simulink model "mcp"  (R2020a)
settings: configuration reference "globalConfig" (kept outside this file)
InitFcn:
  | load pot.mat;
  | load rpm.mat;
undefined symbols (not defined in the file): pot_kw, rpm
settings Model: OrderedModelArguments=off  Creator=victo  LastModifiedBy=ToT_IPMS_03
settings ConfigSetRef: SourceName=globalConfig  SourceLocation=Base Workspace

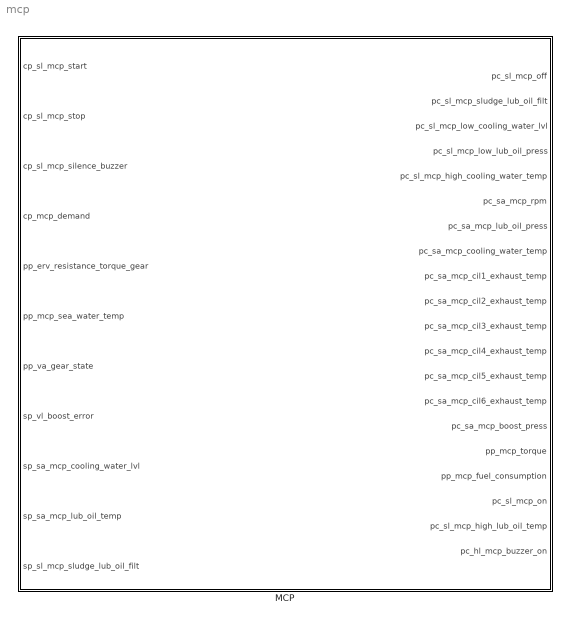
== system mcp ==
  MCP : Subsystem

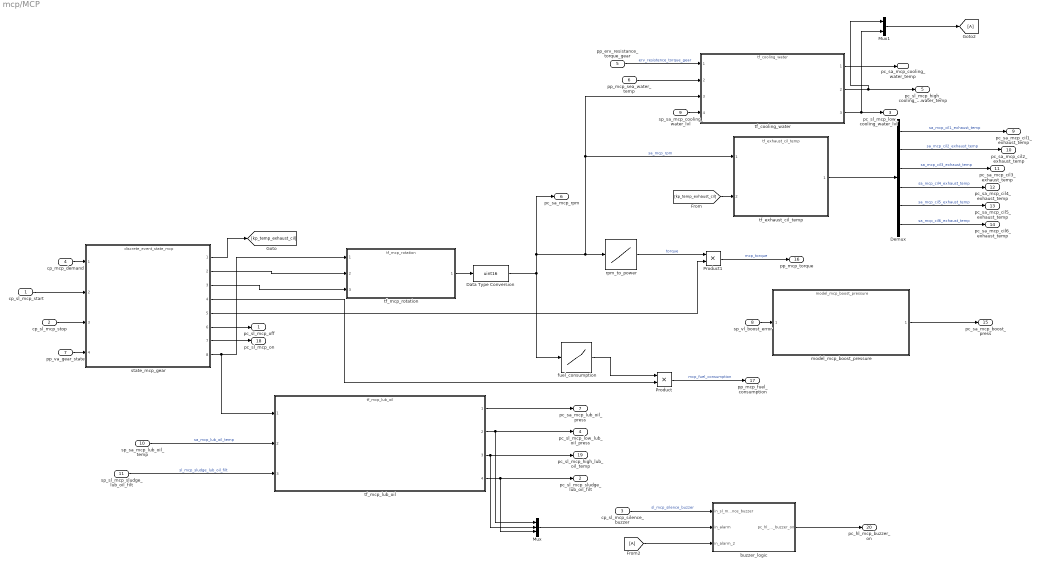
== system mcp/MCP ==
  cp_sl_mcp_start : Inport  OutMin=[0]  OutMax=[1]  OutDataTypeStr=boolean
  cp_sl_mcp_stop : Inport  Port=2  OutMin=[0]  OutMax=[1]  OutDataTypeStr=boolean
  cp_sl_mcp_silence_buzzer : Inport  Port=3  OutMin=[0]  OutMax=[1]  OutDataTypeStr=boolean
  cp_mcp_demand : Inport  Port=4  OutMin=[-100]  OutMax=[100]  OutDataTypeStr=int16  Unit=%
  pp_erv_resistance_torque_gear : Inport  Port=5  OutMin=0  OutMax=1000  OutDataTypeStr=double  Unit=N*m
  pp_mcp_sea_water_temp : Inport  Port=6  OutMin=0  OutMax=90  OutDataTypeStr=uint16  Unit=°C
  pp_va_gear_state : Inport  Port=7  OutMin=0  OutMax=2  OutDataTypeStr=uint8
  sp_vl_boost_error : Inport  Port=8  OutDataTypeStr=boolean
  sp_sa_mcp_cooling_water_lvl : Inport  Port=9  OutMin=[0]  OutMax=[100]  OutDataTypeStr=uint16  Unit=%
  sp_sa_mcp_lub_oil_temp : Inport  Port=10  OutMin=[0]  OutMax=[100]  OutDataTypeStr=uint16  Unit=°C
  sp_sl_mcp_sludge_lub_oil_filt : Inport  Port=11  OutDataTypeStr=boolean
  Data Type Conversion : DataTypeConversion  OutDataTypeStr=uint16
  Demux : Demux  Outputs=6
  Mux : Mux  Inputs=3
  Mux1 : Mux  Inputs=2
  Product : Product
  Product1 : Product
  buzzer_logic : Subsystem
  fuel_consumption : Lookup_n-D  NumberOfTableDimensions=1  BreakpointsForDimension1=[1000,1100,1200,1300,1400,1500,1600,1700,1800,1900]  Table=[25,30,37,45,55,68,82,101,122,145]  ExtrapMethod=Clip  InternalRulePriority=Speed  RndMeth=Simplest  InputSameDT=on
  model_mcp_boost_pressure : ModelReference  ModelNameDialog=model_mcp_boost_pressure  SimulationMode=Normal  ModelReferenceVersion=2.63
  rpm_to_power : Lookup_n-D  NumberOfTableDimensions=1  BreakpointsForDimension1=rpm  Table=pot_kw./rpm  ExtrapMethod=Clip  InternalRulePriority=Speed  RndMeth=Simplest  InputSameDT=on
  state_mcp_gear : ModelReference  ModelNameDialog=discrete_event_state_mcp.slx  SimulationMode=Normal  ModelReferenceVersion=2.44
  tf_cooling_water : ModelReference  ModelNameDialog=tf_cooling_water.slx  SimulationMode=Normal  ModelReferenceVersion=1.16
  tf_exhaust_cil_temp : ModelReference  ModelNameDialog=tf_exhaust_cil_temp.slx  SimulationMode=Normal  ModelReferenceVersion=1.10
  tf_mcp_lub_oil : ModelReference  ModelNameDialog=tf_mcp_lub_oil  SimulationMode=Normal  ModelReferenceVersion=1.29
  tf_mcp_rotation : ModelReference  ModelNameDialog=tf_mcp_rotation.slx  SimulationMode=Normal  ModelReferenceVersion=2.30
  pc_sl_mcp_off : Outport  OutMin=[0]  OutMax=[1]  OutDataTypeStr=boolean
  pc_sl_mcp_sludge_lub_oil_filt : Outport  Port=2  OutMin=[0]  OutMax=[1]  OutDataTypeStr=boolean
  pc_sl_mcp_low_cooling_water_lvl : Outport  Port=3  OutMin=[0]  OutMax=[1]  OutDataTypeStr=boolean
  pc_sl_mcp_low_lub_oil_press : Outport  Port=4  OutMin=[0]  OutMax=[1]  OutDataTypeStr=boolean
  pc_sl_mcp_high_cooling_water_temp : Outport  Port=5  OutMin=[0]  OutMax=[1]  OutDataTypeStr=boolean
  pc_sa_mcp_rpm : Outport  Port=6  OutMin=[0]  OutMax=[2000]  OutDataTypeStr=uint16  Unit=rpm
  pc_sa_mcp_lub_oil_press : Outport  Port=7  OutMin=[0]  OutMax=[100]  OutDataTypeStr=uint16  Unit=MPa
  pc_sa_mcp_cooling_water_temp : Outport  Port=8  OutMin=[0]  OutMax=[90]  OutDataTypeStr=uint16  Unit=°C
  pc_sa_mcp_cil1_exhaust_temp : Outport  Port=9  OutMin=[20]  OutMax=[650]  OutDataTypeStr=uint16  Unit=°C
  pc_sa_mcp_cil2_exhaust_temp : Outport  Port=10  OutMin=[20]  OutMax=[650]  OutDataTypeStr=uint16  Unit=°C
  pc_sa_mcp_cil3_exhaust_temp : Outport  Port=11  OutMin=[20]  OutMax=[650]  OutDataTypeStr=uint16  Unit=°C
  pc_sa_mcp_cil4_exhaust_temp : Outport  Port=12  OutMin=[20]  OutMax=[650]  OutDataTypeStr=uint16  Unit=°C
  pc_sa_mcp_cil5_exhaust_temp : Outport  Port=13  OutMin=[20]  OutMax=[650]  OutDataTypeStr=uint16  Unit=°C
  pc_sa_mcp_cil6_exhaust_temp : Outport  Port=14  OutMin=[20]  OutMax=[650]  OutDataTypeStr=uint16  Unit=°C
  pc_sa_mcp_boost_press : Outport  Port=15  OutMin=[-10]  OutMax=[10]  OutDataTypeStr=int16  Unit=MPa
  pp_mcp_torque : Outport  Port=16
  pp_mcp_fuel_consumption : Outport  Port=17
  pc_sl_mcp_on : Outport  Port=18  OutMin=[0]  OutMax=[1]  OutDataTypeStr=boolean
  pc_sl_mcp_high_lub_oil_temp : Outport  Port=19  OutDataTypeStr=boolean
  pc_hl_mcp_buzzer_on : Outport  Port=20
  wires:
  cp_mcp_demand/1 -> state_mcp_gear/1
  tf_mcp_rotation/1 -> Data Type Conversion/1
  tf_mcp_lub_oil/1 -> pc_sa_mcp_lub_oil_press/1
  fuel_consumption/1 -> Product/1
  Product/1 -> pp_mcp_fuel_consumption/1  "mcp_fuel_consumption"
  rpm_to_power/1 -> Product1/1  "torque"
  Product1/1 -> pp_mcp_torque/1  "mcp_torque"
  Demux/1 -> pc_sa_mcp_cil1_exhaust_temp/1  "sa_mcp_cil1_exhaust_temp"
  Demux/2 -> pc_sa_mcp_cil2_exhaust_temp/1  "sa_mcp_cil2_exhaust_temp"
  Demux/3 -> pc_sa_mcp_cil3_exhaust_temp/1  "sa_mcp_cil3_exhaust_temp"
  Demux/4 -> pc_sa_mcp_cil4_exhaust_temp/1  "sa_mcp_cil4_exhaust_temp"
  Demux/5 -> pc_sa_mcp_cil5_exhaust_temp/1  "sa_mcp_cil5_exhaust_temp"
  Demux/6 -> pc_sa_mcp_cil6_exhaust_temp/1  "sa_mcp_cil6_exhaust_temp"
  [kp_temp_exhaust_cil] -> tf_exhaust_cil_temp/2
  tf_exhaust_cil_temp/1 -> Demux/1
  cp_sl_mcp_stop/1 -> state_mcp_gear/3
  state_mcp_gear/1 -> [kp_temp_exhaust_cil]
  state_mcp_gear/2 -> tf_mcp_rotation/2
  state_mcp_gear/3 -> tf_mcp_rotation/3
  state_mcp_gear/4 -> Product/2
  state_mcp_gear/5 -> Product1/2
  state_mcp_gear/6 -> pc_sl_mcp_off/1
  state_mcp_gear/7 -> pc_sl_mcp_on/1
  pp_mcp_sea_water_temp/1 -> tf_cooling_water/2
  pp_erv_resistance_torque_gear/1 -> tf_cooling_water/1  "erv_resistence_torque_gear"
  tf_cooling_water/1 -> pc_sa_mcp_cooling_water_temp/1
  state_mcp_gear/8 -> tf_mcp_lub_oil/1, tf_mcp_rotation/1
  pp_va_gear_state/1 -> state_mcp_gear/4
  sp_vl_boost_error/1 -> model_mcp_boost_pressure/1
  model_mcp_boost_pressure/1 -> pc_sa_mcp_boost_press/1
  Data Type Conversion/1 -> fuel_consumption/1, pc_sa_mcp_rpm/1, rpm_to_power/1, tf_exhaust_cil_temp/1, tf_cooling_water/3  "sa_mcp_rpm"
  sp_sa_mcp_cooling_water_lvl/1 -> tf_cooling_water/4
  tf_mcp_lub_oil/2 -> Mux/1, pc_sl_mcp_low_lub_oil_press/1
  sp_sa_mcp_lub_oil_temp/1 -> tf_mcp_lub_oil/2  "sa_mcp_lub_oil_temp"
  tf_mcp_lub_oil/3 -> Mux/2, pc_sl_mcp_high_lub_oil_temp/1
  sp_sl_mcp_sludge_lub_oil_filt/1 -> tf_mcp_lub_oil/3  "sl_mcp_sludge_lub_oil_filt"
  tf_mcp_lub_oil/4 -> Mux/3, pc_sl_mcp_sludge_lub_oil_filt/1
  tf_cooling_water/2 -> Mux1/1, pc_sl_mcp_high_cooling_water_temp/1
  tf_cooling_water/3 -> pc_sl_mcp_low_cooling_water_lvl/1, Mux1/2
  Mux1/1 -> [A]
  cp_sl_mcp_silence_buzzer/1 -> buzzer_logic/1(in_sl_mcp_silence_buzzer)  "sl_mcp_silence_buzzer"
  Mux/1 -> buzzer_logic/2(in_alarm)
  [A] -> buzzer_logic/3(in_alarm_2)
  buzzer_logic/1(pc_hl_mcp_buzzer_on) -> pc_hl_mcp_buzzer_on/1
  cp_sl_mcp_start/1 -> state_mcp_gear/2

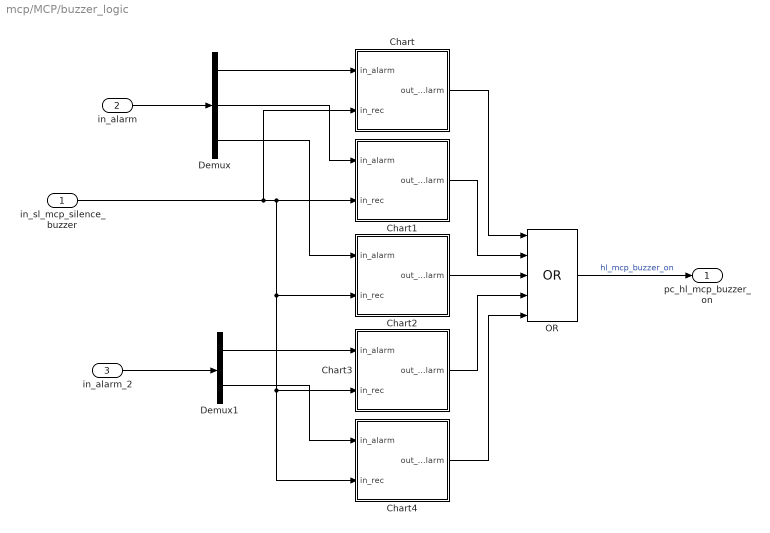
== system mcp/MCP/buzzer_logic ==
  in_sl_mcp_silence_buzzer : Inport  OutDataTypeStr=boolean
  in_alarm : Inport  Port=2  OutDataTypeStr=boolean
  in_alarm_2 : Inport  Port=3
  Chart : Stateflow chart  TreatAsAtomicUnit=on
  Chart1 : Stateflow chart  TreatAsAtomicUnit=on
  Chart2 : Stateflow chart  TreatAsAtomicUnit=on
  Chart3 : Stateflow chart  TreatAsAtomicUnit=on
  Chart4 : Stateflow chart  TreatAsAtomicUnit=on
  Demux : Demux  Outputs=3
  Demux1 : Demux  Outputs=2
  OR : Logic  Operator=OR  Inputs=5  IconShape=distinctive  AllPortsSameDT=off  OutDataTypeStr=boolean
  pc_hl_mcp_buzzer_on : Outport
  wires:
  Chart3/1(out_alarm) -> OR/4
  Chart4/1(out_alarm) -> OR/5
  Demux/1 -> Chart/1(in_alarm)
  Demux/3 -> Chart2/1(in_alarm)
  Chart2/1(out_alarm) -> OR/3
  Chart1/1(out_alarm) -> OR/2
  OR/1 -> pc_hl_mcp_buzzer_on/1  "hl_mcp_buzzer_on"
  Demux/2 -> Chart1/1(in_alarm)
  Demux1/1 -> Chart3/1(in_alarm)
  Demux1/2 -> Chart4/1(in_alarm)
  in_alarm_2/1 -> Demux1/1
  Chart/1(out_alarm) -> OR/1
  in_alarm/1 -> Demux/1
  in_sl_mcp_silence_buzzer/1 -> Chart3/2(in_rec), Chart4/2(in_rec), Chart2/2(in_rec), Chart1/2(in_rec), Chart/2(in_rec)

== stateflow chart mcp/MCP/buzzer_logic/Chart ==
  state OFF
    entry:
    out_alarm=false;
  state Alarmando
    entry:
    out_alarm=true;
  state Reconhecido
    entry:
    out_alarm=false;
  (default) -> OFF
  OFF -> Alarmando : [in_alarm==true]
  Alarmando -> Reconhecido : [in_rec==true]
  Reconhecido -> OFF : [in_alarm==false]
  data: in_alarm input; out_alarm output; in_rec input

== stateflow chart mcp/MCP/buzzer_logic/Chart1 ==
  state OFF
    entry:
    out_alarm=false;
  state Alarmando
    entry:
    out_alarm=true;
  state Reconhecido
    entry:
    out_alarm=false;
  (default) -> OFF
  OFF -> Alarmando : [in_alarm==true]
  Alarmando -> Reconhecido : [in_rec==true]
  Reconhecido -> OFF : [in_alarm==false]
  data: in_alarm input; out_alarm output; in_rec input

== stateflow chart mcp/MCP/buzzer_logic/Chart2 ==
  state OFF
    entry:
    out_alarm=false;
  state Alarmando
    entry:
    out_alarm=true;
  state Reconhecido
    entry:
    out_alarm=false;
  (default) -> OFF
  OFF -> Alarmando : [in_alarm==true]
  Alarmando -> Reconhecido : [in_rec==true]
  Reconhecido -> OFF : [in_alarm==false]
  data: in_alarm input; out_alarm output; in_rec input

== stateflow chart mcp/MCP/buzzer_logic/Chart3 ==
  state OFF
    entry:
    out_alarm=false;
  state Alarmando
    entry:
    out_alarm=true;
  state Reconhecido
    entry:
    out_alarm=false;
  (default) -> OFF
  OFF -> Alarmando : [in_alarm==true]
  Alarmando -> Reconhecido : [in_rec==true]
  Reconhecido -> OFF : [in_alarm==false]
  data: in_alarm input; out_alarm output; in_rec input

== stateflow chart mcp/MCP/buzzer_logic/Chart4 ==
  state OFF
    entry:
    out_alarm=false;
  state Alarmando
    entry:
    out_alarm=true;
  state Reconhecido
    entry:
    out_alarm=false;
  (default) -> OFF
  OFF -> Alarmando : [in_alarm==true]
  Alarmando -> Reconhecido : [in_rec==true]
  Reconhecido -> OFF : [in_alarm==false]
  data: in_alarm input; out_alarm output; in_rec input
